simulink model "RobotController2"  (R2017a)
settings: Solver=VariableStepAuto  StartTime=0.0  StopTime=500.0  RelTol=1e-3
settings Model: Creator=Carapinha  LastModifiedBy=Carapinha

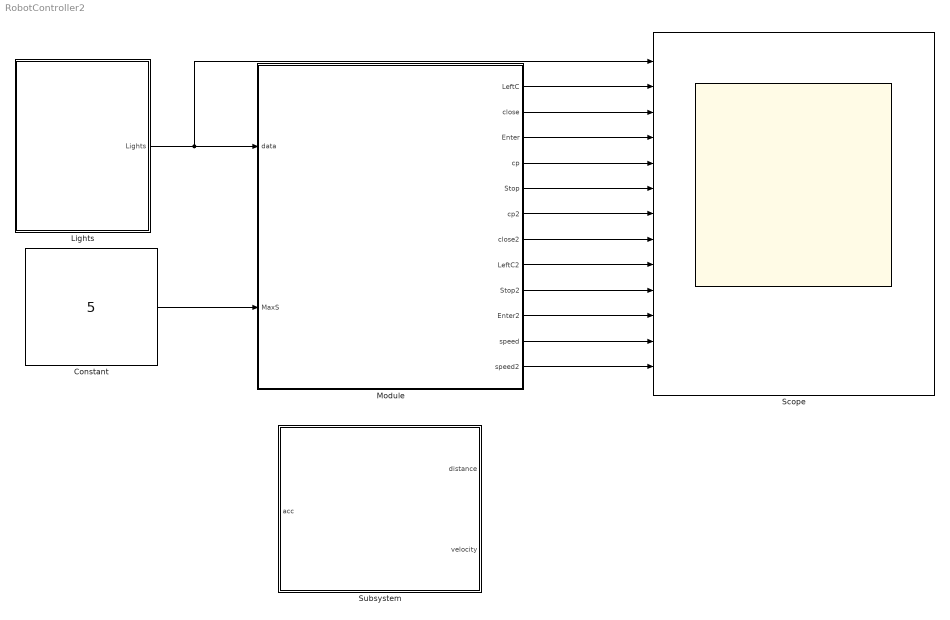
== system RobotController2 ==
  Constant : Constant  Value=5
  Lights : Stateflow chart  TreatAsAtomicUnit=on
  Module : Stateflow chart  TreatAsAtomicUnit=on
  Scope : Scope  NumInputPorts=13
  Subsystem : Subsystem
  wires:
  Module/5(Stop) -> Scope/6
  Module/3(Enter) -> Scope/4
  Constant/1 -> Module/2(MaxS)
  Lights/1(Lights) -> Scope/1, Module/1(data)
  Module/4(cp) -> Scope/5
  Module/1(LeftC) -> Scope/2
  Module/2(close) -> Scope/3
  Module/6(cp2) -> Scope/7
  Module/7(close2) -> Scope/8
  Module/8(LeftC2) -> Scope/9
  Module/9(Stop2) -> Scope/10
  Module/10(Enter2) -> Scope/11
  Module/11(speed) -> Scope/12
  Module/12(speed2) -> Scope/13

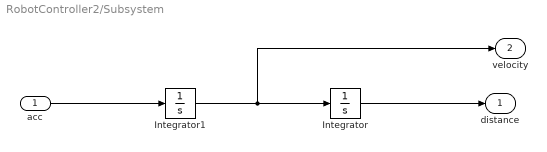
== system RobotController2/Subsystem ==
  acc : Inport
  Integrator : Integrator  InitialCondition=50  WrapState=on  WrappedStateUpperValue=100  WrappedStateLowerValue=0
  Integrator1 : Integrator  InitialCondition=1
  distance : Outport
  velocity : Outport  Port=2
  wires:
  acc/1 -> Integrator1/1
  Integrator1/1 -> velocity/1, Integrator/1
  Integrator/1 -> distance/1

== stateflow chart RobotController2/Lights ==
  state Red
    entry:
    Lights = 0;
  state Green
    entry:
    Lights = 1;
  (default) -> Red
  Green -> Red : [after(0.7, sec)]
  Red -> Green : [after(0.7,sec)]
  data: Lights output

== stateflow chart RobotController2/Module ==
  state Main
    state Robot1 [parallel]
      settings: executionOrder=1
      state move3
        entry:
        LeftC = 0;
        close = 0;
        Enter = 1;
        cp = 0;
        Stop = 0;
      state move1
        entry:
        LeftC = 1;
        close = 0;
        Enter = 0;
        cp = 0;
        Stop = 0;
      state move2
        entry:
        LeftC = 0;
        close = 1;
        Enter = 0;
        cp = 0;
        Stop = 0;
      state Accel
        entry:
        LeftC = 0;
        close = 0;
        Enter = 1;
        cp = 0;
        Stop = 0;
        speed = acc(10);
      state Decel
        entry:
        LeftC = 0;
        close = 0;
        Enter = 0;
        cp = 1;
        Stop = 0;
        speed = acc(-5);
      state Wait
        entry:
        LeftC = 0;
        close = 0;
        Enter = 0;
        cp = 0;
        Stop = 1;
      Main.Robot1.move3 -> Main.Robot1.move1 : [after(0.3,sec)]
      (default) -> Main.Robot1.move1
      Main.Robot1.move1 -> Main.Robot1.move2 : [after(0.3,sec)]
      Main.Robot1.move2 -> Main.Robot1.move3 [order 1] : [Permission1 == 1]
      Main.Robot1.Accel -> Main.Robot1.move3 : [speed == MaxS]
      Main.Robot1.move2 -> Main.Robot1.Decel [order 2] : [after(0.3,sec)]
      Main.Robot1.Decel -> Main.Robot1.Accel [order 1] : [Permission1 == 1]
      Main.Robot1.Decel -> Main.Robot1.Wait [order 2] : [speed == 0]
      Main.Robot1.Wait -> Main.Robot1.Accel [order 1] : [Permission1 == 1]
      Main.Robot1.Wait -> Main.Robot1.Wait [order 2] : [Permission1 == 0]
    state Robot2 [parallel]
      settings: executionOrder=3
      state move3
        entry:
        LeftC2 = 0;
        close2 = 0;
        Enter2 = 1;
        cp2 = 0;
        Stop2 = 0;
      state move1
        entry:
        LeftC2 = 1;
        close2 = 0;
        Enter2 = 0;
        cp2 = 0;
        Stop2 = 0;
      state move2
        entry:
        LeftC2 = 0;
        close2 = 1;
        Enter2 = 0;
        cp2 = 0;
        Stop2 = 0;
      state Accel
        entry:
        LeftC2 = 0;
        close2 = 0;
        Enter2 = 1;
        cp2 = 0;
        Stop2 = 0;
        speed2 = acc(10);
      state Decel
        entry:
        LeftC2 = 0;
        close2 = 0;
        Enter2 = 0;
        cp2 = 1;
        Stop2 = 0;
        speed2 = acc(-5);
      state Wait
        entry:
        LeftC2 = 0;
        close2 = 0;
        Enter2 = 0;
        cp2 = 0;
        Stop2 = 1;
      Main.Robot2.move3 -> Main.Robot2.move1 : [after(0.3,sec)]
      (default) -> Main.Robot2.move1
      Main.Robot2.move1 -> Main.Robot2.move2 : [after(0.3,sec)]
      Main.Robot2.move2 -> Main.Robot2.move3 [order 1] : [Permission2 == 1]
      Main.Robot2.Accel -> Main.Robot2.move3 : [speed2 == MaxS]
      Main.Robot2.move2 -> Main.Robot2.Decel [order 2] : [after(0.3,sec)]
      Main.Robot2.Decel -> Main.Robot2.Accel [order 1] : [Permission2 == 1]
      Main.Robot2.Decel -> Main.Robot2.Wait [order 2] : [speed2 == 0]
      Main.Robot2.Wait -> Main.Robot2.Accel [order 1] : [Permission2 == 1]
      Main.Robot2.Wait -> Main.Robot2.Wait [order 2] : [Permission2 == 0]
    state Controller [parallel]
      settings: executionOrder=2
      state Green
        entry:
        Permission1 = 1;
        Permission2 = 0;
      state RobotState
      state RobotState3
      state Red
        entry:
        Permission1 = 0;
        Permission2 = 1;
      RobotState3 -> RobotState : [LeftC == 1 || LeftC2 == 1]
      (default) -> RobotState
      (junction 79) -> Green [order 1] : [data == 1 && Enter2 ~= 1]
      Green -> RobotState3
      RobotState -> (junction 79) : [(close == 1 || Stop == 1) || (close2 == 1 || Stop2 == 1)]
      (junction 79) -> Red [order 2] : [data == 0 && Enter ~= 1]
      Red -> RobotState3
    state SpeedC1 [parallel]
      settings: executionOrder=4
      state Speed1
        entry:
        speed = MaxS;
        Decel = 1;
        Accel = 0;
      state Speed6
        entry:
        speed = 0;
        Decel = 0;
        Accel = 1;
      state Speed2
        entry:
        speed = 4;
      state Speed4
        entry:
        speed = 2;
      state Speed3
        entry:
        speed = 3;
      state Speed5
        entry:
        speed = 1;
      (default) -> Main.SpeedC1.Speed1
      Main.SpeedC1.Speed2 -> Main.SpeedC1.Speed1 [order 2] : [after(1,sec) && Accel == 1]
      Main.SpeedC1.Speed1 -> Main.SpeedC1.Speed2 : [after(1,sec) && Decel == 1 && cp == 1]
      Main.SpeedC1.Speed6 -> Main.SpeedC1.Speed5 : [after(1,sec) && Accel == 1 && Enter == 1]
      Main.SpeedC1.Speed5 -> Main.SpeedC1.Speed6 [order 1] : [after(1,sec) && Decel == 1]
      Main.SpeedC1.Speed3 -> Main.SpeedC1.Speed2 [order 2] : [after(1,sec) && Accel == 1]
      Main.SpeedC1.Speed2 -> Main.SpeedC1.Speed3 [order 1] : [after(1,sec)  && Decel == 1]
      Main.SpeedC1.Speed3 -> Main.SpeedC1.Speed4 [order 1] : [after(1,sec)  && Decel == 1]
      Main.SpeedC1.Speed4 -> Main.SpeedC1.Speed5 [order 1] : [after(1,sec) && Decel == 1]
      Main.SpeedC1.Speed5 -> Main.SpeedC1.Speed4 [order 2] : [after(1,sec) && Accel == 1]
      Main.SpeedC1.Speed4 -> Main.SpeedC1.Speed3 [order 2] : [after(1,sec) && Accel == 1]
    state SpeedC2 [parallel]
      settings: executionOrder=5
      state Speed1
        entry:
        speed2 = MaxS;
        Decel = 1;
        Accel = 0;
      state Speed6
        entry:
        speed2 = 0;
        Decel = 0;
        Accel = 1;
      state Speed2
        entry:
        speed2 = 4;
      state Speed4
        entry:
        speed2 = 2;
      state Speed3
        entry:
        speed2 = 3;
      state Speed5
        entry:
        speed2 = 1;
      (default) -> Main.SpeedC2.Speed1
      Main.SpeedC2.Speed2 -> Main.SpeedC2.Speed1 [order 2] : [after(1,sec) && Accel == 1]
      Main.SpeedC2.Speed1 -> Main.SpeedC2.Speed2 : [after(1,sec) && Decel == 1 && cp2 == 1]
      Main.SpeedC2.Speed6 -> Main.SpeedC2.Speed5 : [after(1,sec) && Accel == 1 && Enter2 == 1]
      Main.SpeedC2.Speed5 -> Main.SpeedC2.Speed6 [order 1] : [after(1,sec) && Decel == 1]
      Main.SpeedC2.Speed3 -> Main.SpeedC2.Speed2 [order 2] : [after(1,sec) && Accel == 1]
      Main.SpeedC2.Speed2 -> Main.SpeedC2.Speed3 [order 1] : [after(1,sec)  && Decel == 1]
      Main.SpeedC2.Speed3 -> Main.SpeedC2.Speed4 [order 1] : [after(1,sec)  && Decel == 1]
      Main.SpeedC2.Speed4 -> Main.SpeedC2.Speed5 [order 1] : [after(1,sec) && Decel == 1]
      Main.SpeedC2.Speed5 -> Main.SpeedC2.Speed4 [order 2] : [after(1,sec) && Accel == 1]
      Main.SpeedC2.Speed4 -> Main.SpeedC2.Speed3 [order 2] : [after(1,sec) && Accel == 1]
  (default) -> Main
  data: data input; LeftC output; close output; Enter output; cp output; Stop output; MaxS input; cp2 output; Permission1 local; Permission2 local; close2 output; LeftC2 output; Stop2 output; Enter2 output; Decel local; Accel local; speed output; speed2 output
